simulink model "controlled"  (R2020b)
settings: Solver=VariableStepAuto  StartTime=0.0  StopTime=5*orbit.T  RelTol=1e-3
libraries: library x4
settings Model: SimulationMode=accelerator  Creator=loren  LastModifiedBy=loren

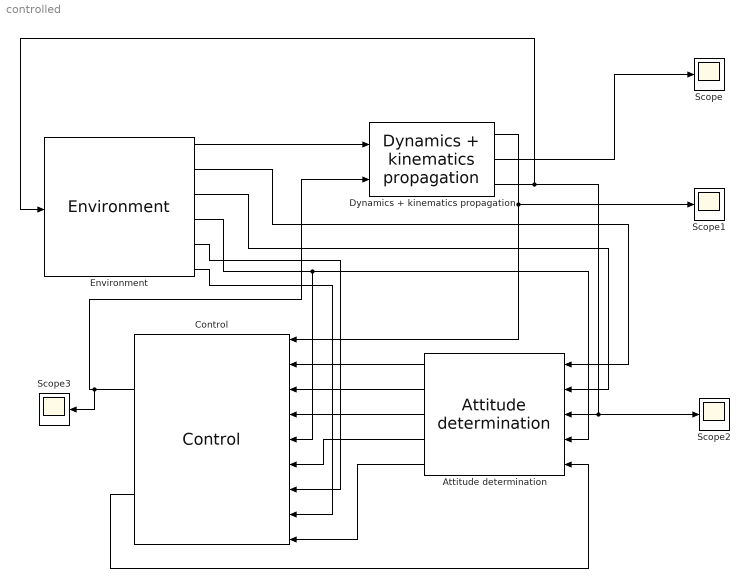
== system controlled ==
  Attitude determination : library/Attitude determination  SystemSampleTime=-1  VariantActivationTime=update diagram  Latency=0  AutoFrameSizeCalculation=off
  Control : library/Control  SystemSampleTime=-1  VariantActivationTime=update diagram  Latency=0  AutoFrameSizeCalculation=off
  Dynamics + kinematics propagation : library/Dynamics + kinematics propagation  SystemSampleTime=-1  VariantActivationTime=update diagram  Latency=0  AutoFrameSizeCalculation=off
  Environment : library/Environment  SystemSampleTime=-1  VariantActivationTime=update diagram  Latency=0  AutoFrameSizeCalculation=off
  Scope{,1..3} (4 alike) : Scope
  wires:
  Environment/1 -> Dynamics + kinematics propagation/1
  Control/1 -> Scope3/1, Dynamics + kinematics propagation/2
  Dynamics + kinematics propagation/3 -> Environment/1, Attitude determination/3, Scope2/1
  Environment/2 -> Attitude determination/1
  Environment/3 -> Attitude determination/2
  Environment/4 -> Attitude determination/4, Control/5
  Control/2 -> Attitude determination/5
  Dynamics + kinematics propagation/1 -> Control/1, Scope1/1
  Attitude determination/1 -> Control/2
  Dynamics + kinematics propagation/2 -> Scope/1
  Attitude determination/5 -> Control/9
  Attitude determination/2 -> Control/3
  Attitude determination/3 -> Control/4
  Attitude determination/4 -> Control/6
  Environment/5 -> Control/7
  Environment/6 -> Control/8
